simulink library "Lib_Thermo_IsentropicCompression_TMATS"  (R2019b)
settings: Solver=ode45  StartTime=0.0  StopTime=10.0  RelTol=1e-3  EnableMultiTasking=on
libraries: Lib_Thermo_Temp2Enth_TMATS x2, Lib_Thermo_Enth2Temp_TMATS x1, Lib_Thermo_PT2S_TMATS x1, Lib_Thermo_SP2T_TMATS x1
Description:
  | Thomas Modules
settings Model: Creator=jwchapm2  LastModifiedBy=bhisma
settings DataIOCC: LimitDataPoints=on  SaveFormat=Array  ReturnWorkspaceOutputs=off
settings OptimizationCC: ExpressionDepthLimit=2147483647  LifeSpan=inf
settings DebuggingCC: UnderspecifiedInitializationDetection=Classic  MergeDetectMultiDrivingBlocksExec=none  SolverPrmCheckMsg=warning  StateNameClashWarn=warning  SFUnexpectedBacktrackingDiag=warning  SFNoUnconditionalDefaultTransitionDiag=warning  SFExecutionAtInitializationDiag=none  ArithmeticOperatorsInVariantConditions=warning
settings HardwareCC: ProdBitPerPointer=32  ProdBitPerSizeT=32  ProdBitPerPtrDiffT=32  ProdLargestAtomicFloat=None  ProdIntDivRoundTo=Undefined  ProdEndianess=Unspecified  ProdWordSize=32  ProdHWDeviceType=32-bit Generic
settings ModelReferenceCC: PropagateSignalLabelsOutOfModel=off
settings SFSimCC: SimUseLocalCustomCode=off  CustomCodeUndefinedFunction=UseInterfaceOnly
settings RTWCC: RTWUseLocalCustomCode=off
settings CodeAppCC: StateflowObjectComments=on
settings GRTTargetCC: TargetLangStandard=C89/C90 (ANSI)  GeneratePreprocessorConditionals=Disable all
settings ConfigComp: CovMetricSettings=dw  CovHtmlReporting=on  CovSaveCumulativeToWorkspaceVar=on  CovSaveSingleToWorkspaceVar=on  CovExternalEMLEnable=off

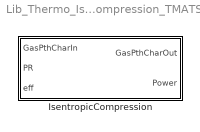
== system Lib_Thermo_IsentropicCompression_TMATS ==
  IsentropicCompression : Subsystem  mask(T-MATS: Isentropic Compression Library Block){}
      mask help: This block performs an isentropic compression on a gas.
      mask Help: web(which('Thermo_TMATS_IsoComp.html'),'-helpbrowser')

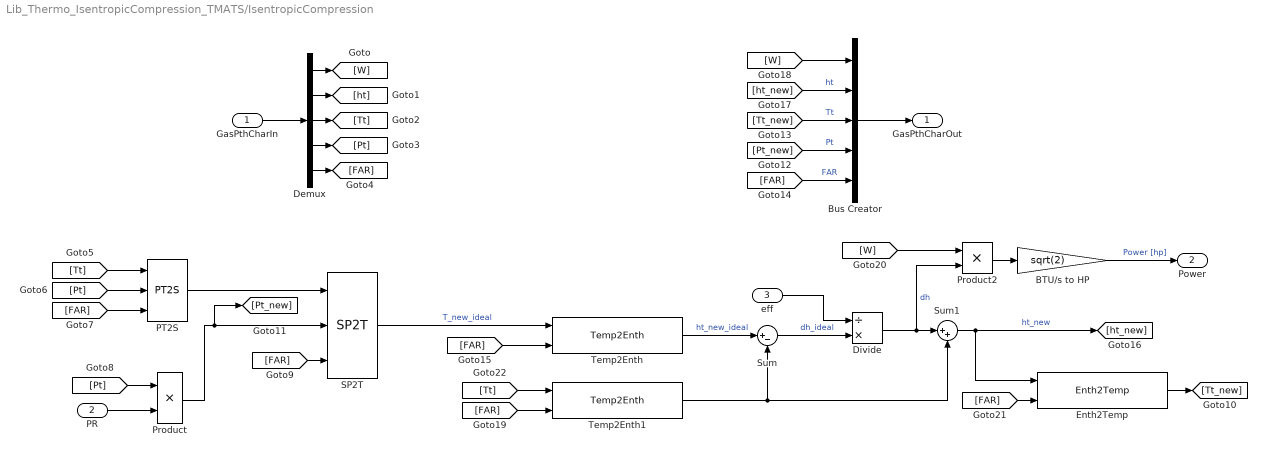
== system Lib_Thermo_IsentropicCompression_TMATS/IsentropicCompression ==
  GasPthCharIn : Inport
  PR : Inport  Port=2
  eff : Inport  Port=3
  BTU/s to HP : Gain  Gain=sqrt(2)
  Bus Creator : BusCreator  Inputs=5
  Demux : Demux  Outputs=5
  Divide : Product  Inputs=/*
  Enth2Temp : Lib_Thermo_Enth2Temp_TMATS/Enth2Temp
  PT2S : Lib_Thermo_PT2S_TMATS/PT2S
  Product : Product
  Product2 : Product
  SP2T : Lib_Thermo_SP2T_TMATS/SP2T
  Sum : Sum  Inputs=|+-
  Sum1 : Sum  Inputs=|++
  Temp2Enth : Lib_Thermo_Temp2Enth_TMATS/Temp2Enth
  Temp2Enth1 : Lib_Thermo_Temp2Enth_TMATS/Temp2Enth
  GasPthCharOut : Outport
  Power : Outport  Port=2
  wires:
  [FAR] -> Bus Creator/5  "FAR"
  [Tt_new] -> Bus Creator/3  "Tt"
  SP2T/1 -> Temp2Enth/1  "T_new_ideal"
  [FAR] -> SP2T/3
  PR/1 -> Product/2
  [W] -> Bus Creator/1
  Temp2Enth/1 -> Sum/1  "ht_new_ideal"
  [FAR] -> Temp2Enth/2
  [Pt] -> Product/1
  Enth2Temp/1 -> [Tt_new]
  Product/1 -> [Pt_new], SP2T/2
  [ht_new] -> Bus Creator/2  "ht"
  Sum/1 -> Divide/2  "dh_ideal"
  [Pt_new] -> Bus Creator/4  "Pt"
  Temp2Enth1/1 -> Sum1/2, Sum/2
  Sum1/1 -> Enth2Temp/1, [ht_new]  "ht_new"
  [FAR] -> Enth2Temp/2
  eff/1 -> Divide/1
  [Tt] -> PT2S/1
  Divide/1 -> Product2/2, Sum1/1  "dh"
  [FAR] -> PT2S/3
  [Pt] -> PT2S/2
  GasPthCharIn/1 -> Demux/1
  PT2S/1 -> SP2T/1
  Bus Creator/1 -> GasPthCharOut/1
  Demux/2 -> [ht]
  Demux/1 -> [W]
  Demux/3 -> [Tt]
  Demux/5 -> [FAR]
  Demux/4 -> [Pt]
  [W] -> Product2/1
  Product2/1 -> BTU/s to HP/1
  BTU/s to HP/1 -> Power/1  "Power [hp]"
  [FAR] -> Temp2Enth1/2
  [Tt] -> Temp2Enth1/1
